simulink model "Capstone_MPC_Final"  (R2024b)
settings: Solver=ode4  StartTime=0.0  StopTime=tsim  FixedStep=baseRate  RelTol=1e-6  AbsTol=1e-6
values from neighbouring files (symbols this model uses):
  C = [cos(theta), -sin(theta) ... (first row only)    [Run_Initializer.m]
  docking_face = [0 1]'    [Run_Initializer.m]
  docking_offset = [0 0 0]'    [Run_Initializer.m]
  eta = 0.2    [Run_Initializer.m]
  F_t = [kron(eye(N_h),  [zeros(2,3), eye(2), zeros(2,4)]) ... (first row only)    [Run_Initializer.m]
  f_t = [kron(ones(N_h, 1), [xLength yLength]' - edge_buffer) ... (first row only)    [Run_Initializer.m]
  F_u = [kron(eye(N_h),  [eye(3), zeros(3,6)]) ... (first row only)    [Run_Initializer.m]
  f_u = kron(ones(2*N_h, 1), u_max')    [Run_Initializer.m]
  F_v = [kron(eye(N_h),  [zeros(1,5), 1, zeros(1,3)]) ... (first row only)    [Run_Initializer.m]
  gamma = 0.95    [Run_Initializer.m]
  Gamma1_el = 0.12    [Run_Initializer.m]
  Gamma1_sh = 0.005    [Run_Initializer.m]
  Gamma1_wr = 0.025    [Run_Initializer.m]
  Gamma2_el = 5    [Run_Initializer.m]
  Gamma2_sh = 5    [Run_Initializer.m]
  Gamma2_wr = 5    [Run_Initializer.m]
  Gamma3_el = 10    [Run_Initializer.m]
  Gamma3_sh = 40    [Run_Initializer.m]
  Gamma3_wr = 40    [Run_Initializer.m]
  Gamma4_el = 0.039    [Run_Initializer.m]
  Gamma4_sh = 0.015    [Run_Initializer.m]
  Gamma4_wr = 0.029    [Run_Initializer.m]
  Gamma5_el = 800    [Run_Initializer.m]
  Gamma5_sh = 800    [Run_Initializer.m]
  Gamma5_wr = 800    [Run_Initializer.m]
  Gamma6_el = 0.000001    (= 1e-06)    [Run_Initializer.m]
  Gamma6_sh = 0.005    [Run_Initializer.m]
  Gamma6_wr = 0.02    [Run_Initializer.m]
  H = kron(eye(N_h), [R, zeros(3,6); zeros(6,3), Q])    [Run_Initializer.m]
  Kd_elarm = 0.8    [Run_Initializer.m]
  Kd_sharm = 1.0    (= 1)    [Run_Initializer.m]
  Kd_wrarm = 0.6    [Run_Initializer.m]
  Kp_elarm = 1.2    [Run_Initializer.m]
  Kp_sharm = 1.5    [Run_Initializer.m]
  Kp_wrarm = 1.0    (= 1)    [Run_Initializer.m]
  lambda = (alpha^2)*(6 + kappa) - 6    (= 15.06)    [Run_Initializer.m]
  lidar_FOV = 40*d2r    (= 0.698131700798)    [Run_Initializer.m]
  lidar_offset = [0.145, 0.087]'    [Run_Initializer.m]
  PWMFreq = 5    [Run_Initializer.m]
  Q_k = [1e-6*eye(3)  zeros(3,3) ... (first row only)    [Run_Initializer.m]
  r_hold_min = [0.8; (0.3+0.05)]    [Run_Initializer.m]
  R_k = diag([0.02^2 0.02^2 0.01^2])    [Run_Initializer.m]
  T_d = 2    [Run_Initializer.m]
  Tz_lim_elarm = .1    (= 0.1)    [Run_Initializer.m]
  Tz_lim_sharm = .1    (= 0.1)    [Run_Initializer.m]
  Tz_lim_wrarm = .1    (= 0.1)    [Run_Initializer.m]
  w_c = [w_c0, w_i.*ones(1, 2*6)]    [Run_Initializer.m]
  w_m = [w_m0, w_i.*ones(1, 2*6)]    [Run_Initializer.m]
  x_BLACK_0 = [(1/3)*xLength (1/3)*yLength-0.2 280*d2r 0.01 0.005 1.88*d2r]'    [Run_Initializer.m]
  x_RED_0 = [3.2 2.1 0 0 0 0]'    [Run_Initializer.m]
  zeta = 10*d2r    (= 0.174532925199)    [Run_Initializer.m]
undefined symbols (not defined in the file or in its folder): a1, a2, a3, b0, b1, b2, b3, baseRate, dataRate, DiscIntNeverNeededParam, drop_states_ARM, drop_states_BLACK, drop_states_BLUE, drop_states_RED, F_black_X_nominal, F_black_Y_nominal, F_blue_X_nominal, F_blue_Y_nominal, F_red_X_nominal, F_red_Y_nominal, F_thrusters_BLACK, F_thrusters_BLUE, F_thrusters_RED, home_states_BLACK, home_states_BLUE, home_states_RED, IBLACK, IBLUE, IDIST, IEE, init_states_BLACK, init_states_BLUE, init_states_RED, IPROX, IRED, K_BLACK, K_BLUE, K_RED, Kd_tb, Kd_tblue, Kd_tr, Kd_xb, Kd_xblue, Kd_xr, Kd_yb, Kd_yblue, Kd_yr, Kp_tb, Kp_tblue, Kp_tr, Kp_xb, Kp_xblue, Kp_xr, Kp_yb, Kp_yblue, Kp_yr, mBLACK, mBLUE, mDIST, mEE ... (+21)
libraries: simulink x30, nvidiaSharedBlocks x18, MainLibrary x5, dspsigops x4, dspstat3 x3, dspinverses x3, dspmathops x1, nvidiaIMUSensorslib x1
(part 2 of 8)

== system Capstone_MPC_Final/Gyro.//Accel. Code ==
  Data Store Read1 : DataStoreRead  DataStoreName=isSim  IndexOptions=Index vector (dialog)  Indices=1  OutputSizes=1
  Log Gyro/Accel : Subsystem  TreatAsAtomicUnit=on
  This IF block determines whether or not to run the exp code : If  IfExpression=u1 == 0  ShowElse=off
  wires:
  This IF block determines whether or not to run the exp code/1 -> Log Gyro/Accel/Action
  Data Store Read1/1 -> This IF block determines whether or not to run the exp code/1

== system Capstone_MPC_Final/LiDAR Camera Code ==
  Check Measurement : MATLAB Function  TreatAsAtomicUnit=on
  Data Store Write : DataStoreWrite  DataStoreName=LiDAR_Data  IndexOptions=Index vector (dialog)  Indices=1  OutputSizes=1
  Data Type Conversion : DataTypeConversion  SaturateOnIntegerOverflow=off  RndMeth=Floor
  Delay : Delay  DelayLength=1  InitialCondition=0
  Demux : Demux  Outputs=[8,1]
  Equal : RelationalOperator  Operator=~=  OutDataTypeStr=boolean  RndMeth=Simplest  InputSameDT=off
  Get Real Measurement : Subsystem
  Get Simulated Measurement : Subsystem
  If : If
  Recieve Computer Vision Data : nvidiaSharedBlocks/UDP Receive  localURL='0.0.0.0'  localPort=43002  remoteURL='0.0.0.0'  remotePort=-1  recvBufferSize=8192  signalDatatype=single  dims=9  isVarSize=off  showBlockingTime=off  blockingTime=0  sampletime=-1  blockPlatform=NVIDIA
  Reshape : Reshape  OutputDimensionality=Customize  OutputDimensions=[9,1]
  Simulate Measurements : Constant  Value=0  OutDataTypeStr=Inherit: Inherit via back propagation
  Terminator : Terminator
  wires:
  If/1 -> Get Simulated Measurement/Action
  Simulate Measurements/1 -> If/1
  If/2 -> Get Real Measurement/Action
  Recieve Computer Vision Data/1 -> Data Type Conversion/1
  Data Type Conversion/1 -> Reshape/1
  Recieve Computer Vision Data/2 -> Terminator/1
  Equal/1 -> Check Measurement/2(new)
  Demux/1 -> Check Measurement/1("z ")
  Reshape/1 -> Demux/1
  Demux/2 -> Equal/2, Delay/1
  Delay/1 -> Equal/1
  Check Measurement/1(z) -> Data Store Write/1

== system Capstone_MPC_Final/Manipulator Encoder Data ==
  note: This if statement checks if a simulation is being performed. If not, it also checks that this code is being run on the RED platform. If it is, then the arm encoders are used to collect the joint angles. NOTE, the encoder data is collected very slowly, about 0.5 Hz. When the diagram is running faster then this collection rate, previous values of the encoder are held constant.
  Change ARM Behavior : Subsystem  TreatAsAtomicUnit=on
  Data Store Read1 : DataStoreRead  DataStoreName=WhoAmI  IndexOptions=Index vector (dialog)  Indices=1  OutputSizes=1
  Data Store Read2 : DataStoreRead  DataStoreName=isSim  IndexOptions=Index vector (dialog)  Indices=1  OutputSizes=1
  "This IF block determines whether or not to run the RED sim/exp " : If  NumInputs=2  IfExpression=u1 == 1 & u2 == 0  ShowElse=off
  wires:
  Data Store Read2/1 -> "This IF block determines whether or not to run the RED sim/exp "/2
  "This IF block determines whether or not to run the RED sim/exp "/1 -> Change ARM Behavior/Action
  Data Store Read1/1 -> "This IF block determines whether or not to run the RED sim/exp "/1

== system Capstone_MPC_Final/Model Predictive Control ==
  Enable : EnablePort
  Clock : Clock
  Data Store Write : DataStoreWrite  DataStoreName=Shutoff_Time  IndexOptions=Index vector (dialog)  Indices=1  OutputSizes=1
  Model Predictive Control : Subsystem  TreatAsAtomicUnit=on  SystemSampleTime=T_d
  Unscented Kalman Filter : Subsystem  TreatAsAtomicUnit=on  SystemSampleTime=baseRate
  wires:
  Clock/1 -> Data Store Write/1

== system Capstone_MPC_Final/PhaseSpace Camera Code ==
  note: In this subsection, the "if" statement is used to determine if this is a simulation or not. If it is not a simulation, then code is run to receive PhaseSpace camera data via UDP. The PhaseSpace code is currently a standalone executable that should not need to be modified by most users. The code sends all data for all platforms to each platform near simultaneously. If this is a simulation, then no data is required, but a continuous clock is created.
  Data Store Read2 : DataStoreRead  DataStoreName=isSim  IndexOptions=Index vector (dialog)  Indices=1  OutputSizes=1
  "If performing an experiment, grab the PhaseSpace data. Otherwise, use a clock to set time in SIM." : If  IfExpression=u1 == 0  ElseIfExpressions=u1 == 1  ShowElse=off
  Initialize Universal Time (Simulation) : Subsystem  TreatAsAtomicUnit=on
  Use Hardware to Obtain States : Subsystem  TreatAsAtomicUnit=on
  wires:
  Data Store Read2/1 -> "If performing an experiment, grab the PhaseSpace data. Otherwise, use a clock to set time in SIM."/1
  "If performing an experiment, grab the PhaseSpace data. Otherwise, use a clock to set time in SIM."/2 -> Initialize Universal Time (Simulation)/Action
  "If performing an experiment, grab the PhaseSpace data. Otherwise, use a clock to set time in SIM."/1 -> Use Hardware to Obtain States/Action

== system Capstone_MPC_Final/Platform Identification ==
  Data Store Read1 : DataStoreRead  DataStoreName=isSim  IndexOptions=Index vector (dialog)  Indices=1  OutputSizes=1
  "If 'simMode' set to '1', then this is a simulation and the dynamics will be simulated. Otherwise, this is an experiment, and the simulation will not be run." : If  IfExpression=u1 == 0  ShowElse=off
  Subsystem : Subsystem
  wires:
  "If 'simMode' set to '1', then this is a simulation and the dynamics will be simulated. Otherwise, this is an experiment, and the simulation will not be run."/1 -> Subsystem/Action
  Data Store Read1/1 -> "If 'simMode' set to '1', then this is a simulation and the dynamics will be simulated. Otherwise, this is an experiment, and the simulation will not be run."/1

== system Capstone_MPC_Final/Robotic Arm Code ==
  note: In this subsection, the "if" statements are used to determine two things: 1) whether or not a simulation is begin performed,
      | then 2) if an experiment is being performed, then which platform is the diagram compiled on. The "IdentifyPlatform" variable
      | is obtained using a custom C++ function which gets the computer name for each platform. NOTE that the arm code only runs on RED.
  Change ARM Behavior : Subsystem  TreatAsAtomicUnit=on
  Data Store Read : DataStoreRead  DataStoreName=WhoAmI  IndexOptions=Index vector (dialog)  Indices=1  OutputSizes=1
  Data Store Read1 : DataStoreRead  DataStoreName=isSim  IndexOptions=Index vector (dialog)  Indices=1  OutputSizes=1
  "This IF block determines whether or not to run the RED sim/exp " : If  NumInputs=2  IfExpression=u1 == 1 & u2 == 0  ShowElse=off
  wires:
  "This IF block determines whether or not to run the RED sim/exp "/1 -> Change ARM Behavior/Action
  Data Store Read1/1 -> "This IF block determines whether or not to run the RED sim/exp "/2
  Data Store Read/1 -> "This IF block determines whether or not to run the RED sim/exp "/1

== system Capstone_MPC_Final/Send Data to Orin ==
  Data Store Read1 : DataStoreRead  DataStoreName=isSim  IndexOptions=Index vector (dialog)  Indices=1  OutputSizes=1
  "If 'simMode' set to '1', then this is a simulation and the dynamics will be simulated. Otherwise, this is an experiment, and the simulation will not be run." : If  IfExpression=u1 == 0  ShowElse=off
  Subsystem : Subsystem
  wires:
  "If 'simMode' set to '1', then this is a simulation and the dynamics will be simulated. Otherwise, this is an experiment, and the simulation will not be run."/1 -> Subsystem/Action
  Data Store Read1/1 -> "If 'simMode' set to '1', then this is a simulation and the dynamics will be simulated. Otherwise, this is an experiment, and the simulation will not be run."/1

== system Capstone_MPC_Final/Simulate Plant Dynamics ==
  Action Port : ActionPort  ActionPortLabel=if(u1 == 1)
  BLACK Dynamics : Subsystem
  BLUE Dynamics : Subsystem
  RED and ARM Dynamics : Subsystem

== system Capstone_MPC_Final/Simulation Status ==
  Constant : Constant  Value=simMode  SampleTime=-1
  Data Store Write : DataStoreWrite  DataStoreName=isSim  IndexOptions=Index vector (dialog)  Indices=1  OutputSizes=1
  wires:
  Constant/1 -> Data Store Write/1

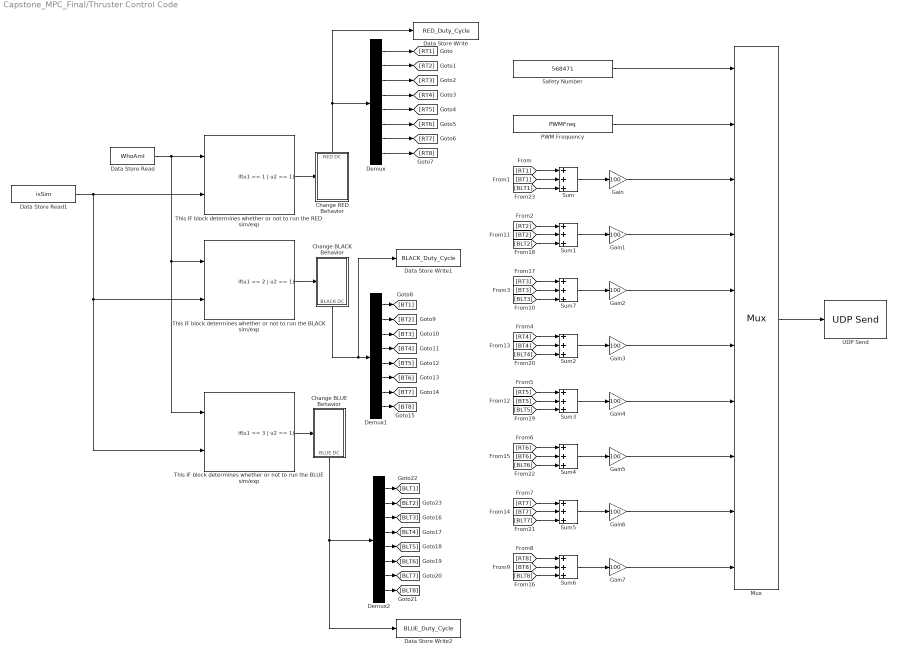
== system Capstone_MPC_Final/Thruster Control Code ==
  Change BLACK Behavior : Subsystem  TreatAsAtomicUnit=on
  Change BLUE Behavior : Subsystem  TreatAsAtomicUnit=on
  Change RED Behavior : Subsystem  TreatAsAtomicUnit=on
  Data Store Read : DataStoreRead  DataStoreName=WhoAmI  IndexOptions=Index vector (dialog)  Indices=1  OutputSizes=1
  Data Store Read1 : DataStoreRead  DataStoreName=isSim  IndexOptions=Index vector (dialog)  Indices=1  OutputSizes=1
  Data Store Write : DataStoreWrite  DataStoreName=RED_Duty_Cycle  IndexOptions=Index vector (dialog)  Indices=1  OutputSizes=1
  Data Store Write1 : DataStoreWrite  DataStoreName=BLACK_Duty_Cycle  IndexOptions=Index vector (dialog)  Indices=1  OutputSizes=1
  Data Store Write2 : DataStoreWrite  DataStoreName=BLUE_Duty_Cycle  IndexOptions=Index vector (dialog)  Indices=1  OutputSizes=1
  Demux : Demux  Outputs=8
  Demux1 : Demux  Outputs=8
  Demux2 : Demux  Outputs=8
  Gain{,1..7} (8 alike) : Gain  Gain=100
  Mux : Mux  Inputs=10
  PWM Frequency : Constant  Value=PWMFreq
  Safety Number : Constant  Value=568471
  Sum{,1..7} (8 alike) : Sum  Inputs=+++
  This IF block determines whether or not to run the BLACK sim/exp : If  NumInputs=2  IfExpression=u1 == 2 | u2 == 1  ShowElse=off
  This IF block determines whether or not to run the BLUE sim/exp : If  NumInputs=2  IfExpression=u1 == 3 | u2 == 1  ShowElse=off
  "This IF block determines whether or not to run the RED sim/exp " : If  NumInputs=2  IfExpression=u1 == 1 | u2 == 1  ShowElse=off
  UDP Send : nvidiaSharedBlocks/UDP Send  remoteURL='127.0.0.1'  remotePort=48291  localURL='0.0.0.0'  localPortSource=Automatically determine  localPort=-1  sampletime=-1  blockPlatform=NVIDIA  separateLengthPort=0
  wires:
  Data Store Read1/1 -> This IF block determines whether or not to run the BLACK sim/exp/2, This IF block determines whether or not to run the BLUE sim/exp/2, "This IF block determines whether or not to run the RED sim/exp "/2
  "This IF block determines whether or not to run the RED sim/exp "/1 -> Change RED Behavior/Action
  This IF block determines whether or not to run the BLACK sim/exp/1 -> Change BLACK Behavior/Action
  Change RED Behavior/1(RED DC) -> Demux/1, Data Store Write/1
  Demux/1 -> [RT1]
  Demux/2 -> [RT2]
  Demux/3 -> [RT3]
  Demux/4 -> [RT4]
  Demux/5 -> [RT5]
  Demux/6 -> [RT6]
  Demux/7 -> [RT7]
  Demux/8 -> [RT8]
  Demux1/5 -> [BT5]
  Demux1/4 -> [BT4]
  Demux1/1 -> [BT1]
  Demux1/8 -> [BT8]
  Demux1/2 -> [BT2]
  Demux1/7 -> [BT7]
  Demux1/6 -> [BT6]
  Demux1/3 -> [BT3]
  Change BLACK Behavior/1(BLACK DC) -> Demux1/1, Data Store Write1/1
  Data Store Read/1 -> This IF block determines whether or not to run the BLUE sim/exp/1, This IF block determines whether or not to run the BLACK sim/exp/1, "This IF block determines whether or not to run the RED sim/exp "/1
  This IF block determines whether or not to run the BLUE sim/exp/1 -> Change BLUE Behavior/Action
  Demux2/5 -> [BLT5]
  Demux2/8 -> [BLT8]
  Demux2/7 -> [BLT7]
  Demux2/2 -> [BLT2]
  Change BLUE Behavior/1(BLUE DC) -> Data Store Write2/1, Demux2/1
  Demux2/1 -> [BLT1]
  Demux2/4 -> [BLT4]
  Demux2/3 -> [BLT3]
  Demux2/6 -> [BLT6]
  [BT5] -> Sum3/2
  [RT4] -> Sum2/1
  Sum3/1 -> Gain4/1
  [RT2] -> Sum1/1
  [BLT4] -> Sum2/3
  [BT3] -> Sum7/2
  [RT5] -> Sum3/1
  PWM Frequency/1 -> Mux/2
  Gain3/1 -> Mux/6
  [BT8] -> Sum6/2
  Gain7/1 -> Mux/10
  Sum6/1 -> Gain7/1
  Sum7/1 -> Gain2/1
  [BT4] -> Sum2/2
  [RT7] -> Sum5/1
  [BLT3] -> Sum7/3
  Gain1/1 -> Mux/4
  Gain/1 -> Mux/3
  [BLT5] -> Sum3/3
  Sum1/1 -> Gain1/1
  Sum2/1 -> Gain3/1
  Gain4/1 -> Mux/7
  [BLT6] -> Sum4/3
  [BT6] -> Sum4/2
  [BT2] -> Sum1/2
  [BLT2] -> Sum1/3
  [RT1] -> Sum/1
  Sum/1 -> Gain/1
  [BT7] -> Sum5/2
  Gain6/1 -> Mux/9
  [BLT7] -> Sum5/3
  [RT8] -> Sum6/1
  [RT6] -> Sum4/1
  Mux/1 -> UDP Send/1
  [BLT8] -> Sum6/3
  [BT1] -> Sum/2
  Sum5/1 -> Gain6/1
  Gain5/1 -> Mux/8
  Sum4/1 -> Gain5/1
  [BLT1] -> Sum/3
  Safety Number/1 -> Mux/1
  [RT3] -> Sum7/1
  Gain2/1 -> Mux/5

== system Capstone_MPC_Final/1 - Experiment Logic/Phase #0: Synchronization ==
  note: Setting the RED thrusters to OFF.
  note: Setting the PUCKS for ALL to OFF.
  note: DISABLE ARM Path Planning.
  note: Setting the BLACK thrusters to OFF.
  note: Setting the BLUE thrusters to OFF.
  note: DISABLE RED Path Planning.
  note: DISABLE BLACK Path Planning.
  note: DISABLE BLUE Path Planning.
  note: DISABLE ARM Control.
  Action Port : ActionPort  ActionPortLabel=if(u1 < u2)
  Constant{1..8} (8 alike) : Constant  Value=0
  Data Store Write : DataStoreWrite  DataStoreName=RED_Control_Law_Enabler  IndexOptions=Index vector (dialog)  Indices=1  OutputSizes=1
  Data Store Write1 : DataStoreWrite  DataStoreName=RED_Logger  IndexOptions=Index vector (dialog)  Indices=1  OutputSizes=1
  Data Store Write2 : DataStoreWrite  DataStoreName=BLACK_Control_Law_Enabler  IndexOptions=Index vector (dialog)  Indices=1  OutputSizes=1
  Data Store Write3 : DataStoreWrite  DataStoreName=BLUE_Control_Law_Enabler  IndexOptions=Index vector (dialog)  Indices=1  OutputSizes=1
  Data Store Write4 : DataStoreWrite  DataStoreName=Float_State  IndexOptions=Index vector (dialog)  Indices=1  OutputSizes=1
  Data Store Write5 : DataStoreWrite  DataStoreName=BLUE_Path_Planner_Selection  IndexOptions=Index vector (dialog)  Indices=1  OutputSizes=1
  Data Store Write6 : DataStoreWrite  DataStoreName=BLACK_Path_Planner_Selection  IndexOptions=Index vector (dialog)  Indices=1  OutputSizes=1
  Data Store Write7 : DataStoreWrite  DataStoreName=RED_Path_Planner_Selection  IndexOptions=Index vector (dialog)  Indices=1  OutputSizes=1
  Data Store Write8 : DataStoreWrite  DataStoreName=ARM_Path_Planner_Selection  IndexOptions=Index vector (dialog)  Indices=1  OutputSizes=1
  Data Store Write9 : DataStoreWrite  DataStoreName=ARM_Control_Law_Enabler  IndexOptions=Index vector (dialog)  Indices=1  OutputSizes=1
  Puck State : Constant  Value=0
  String Constant : StringConstant  String="\"Chaser: Running Phase 0\""
  wires:
  Constant4/1 -> Data Store Write8/1
  Puck State/1 -> Data Store Write4/1
  Constant5/1 -> Data Store Write/1
  Constant1/1 -> Data Store Write2/1
  Constant2/1 -> Data Store Write3/1
  Constant3/1 -> Data Store Write7/1
  Constant6/1 -> Data Store Write6/1
  Constant7/1 -> Data Store Write5/1
  Constant8/1 -> Data Store Write9/1
  String Constant/1 -> Data Store Write1/1

== system Capstone_MPC_Final/1 - Experiment Logic/Phase #1: Start Floating  ==
  note: DISABLE ARM Control.
  note: Setting the BLACK thrusters to OFF.
  note: Setting the PUCKS for ALL to OFF.
  note: DISABLE RED Path Planning.
  note: Setting the RED thrusters to OFF.
  note: Setting the BLUE thrusters to OFF.
  note: DISABLE ARM Path Planning.
  note: DISABLE BLACK Path Planning.
  note: DISABLE BLUE Path Planning.
  Action Port : ActionPort  ActionPortLabel=elseif((u1 < u3 & u1 >= u2))
  Constant{1..8} (8 alike) : Constant  Value=0
  Data Store Write : DataStoreWrite  DataStoreName=RED_Control_Law_Enabler  IndexOptions=Index vector (dialog)  Indices=1  OutputSizes=1
  Data Store Write1 : DataStoreWrite  DataStoreName=RED_Logger  IndexOptions=Index vector (dialog)  Indices=1  OutputSizes=1
  Data Store Write2 : DataStoreWrite  DataStoreName=BLACK_Control_Law_Enabler  IndexOptions=Index vector (dialog)  Indices=1  OutputSizes=1
  Data Store Write3 : DataStoreWrite  DataStoreName=BLUE_Control_Law_Enabler  IndexOptions=Index vector (dialog)  Indices=1  OutputSizes=1
  Data Store Write4 : DataStoreWrite  DataStoreName=Float_State  IndexOptions=Index vector (dialog)  Indices=1  OutputSizes=1
  Data Store Write5 : DataStoreWrite  DataStoreName=BLUE_Path_Planner_Selection  IndexOptions=Index vector (dialog)  Indices=1  OutputSizes=1
  Data Store Write6 : DataStoreWrite  DataStoreName=BLACK_Path_Planner_Selection  IndexOptions=Index vector (dialog)  Indices=1  OutputSizes=1
  Data Store Write7 : DataStoreWrite  DataStoreName=RED_Path_Planner_Selection  IndexOptions=Index vector (dialog)  Indices=1  OutputSizes=1
  Data Store Write8 : DataStoreWrite  DataStoreName=ARM_Path_Planner_Selection  IndexOptions=Index vector (dialog)  Indices=1  OutputSizes=1
  Data Store Write9 : DataStoreWrite  DataStoreName=ARM_Control_Law_Enabler  IndexOptions=Index vector (dialog)  Indices=1  OutputSizes=1
  Puck State : Constant
  String Constant : StringConstant  String="\"Chaser: Running Phase 1\""
  wires:
  Constant7/1 -> Data Store Write5/1
  Constant2/1 -> Data Store Write3/1
  Constant6/1 -> Data Store Write6/1
  Puck State/1 -> Data Store Write4/1
  Constant1/1 -> Data Store Write2/1
  Constant5/1 -> Data Store Write/1
  Constant3/1 -> Data Store Write7/1
  Constant8/1 -> Data Store Write9/1
  Constant4/1 -> Data Store Write8/1
  String Constant/1 -> Data Store Write1/1

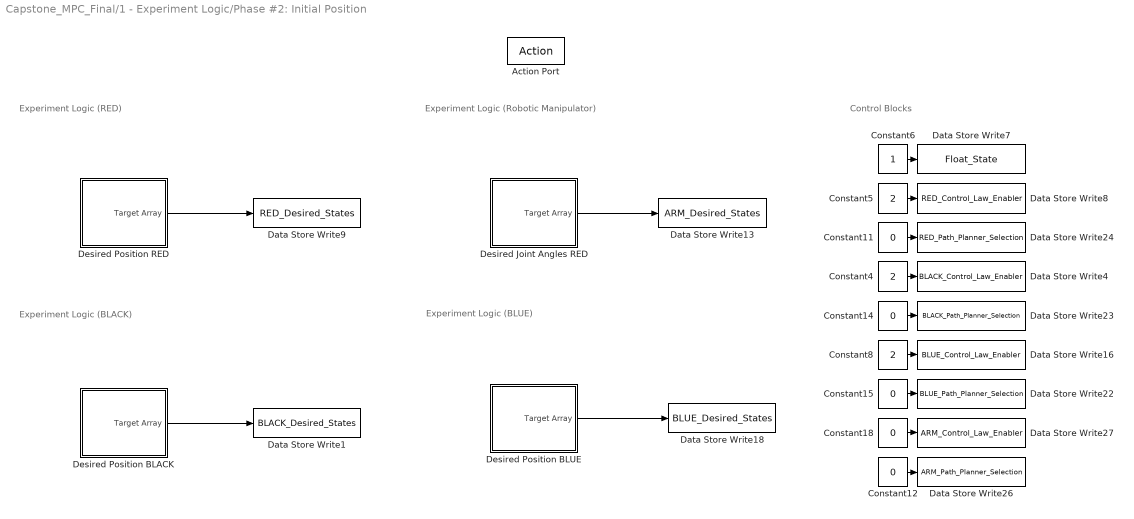
== system Capstone_MPC_Final/1 - Experiment Logic/Phase #2: Initial Position ==
  note: Experiment Logic (BLACK)
  note: Control Blocks
  note: Experiment Logic (RED)
  note: Experiment Logic (Robotic Manipulator)
  note: Experiment Logic (BLUE)
  Action Port : ActionPort  ActionPortLabel=elseif((u1 < u4 & u1 >= u3))
  Constant{11..12,14..15,18} (5 alike) : Constant  Value=0
  Constant4 : Constant  Value=2
  Constant5 : Constant  Value=2
  Constant6 : Constant
  Constant8 : Constant  Value=2
  Data Store Write1 : DataStoreWrite  DataStoreName=BLACK_Desired_States  IndexOptions=Index vector (dialog)  Indices=1  OutputSizes=1
  Data Store Write13 : DataStoreWrite  DataStoreName=ARM_Desired_States  IndexOptions=Index vector (dialog)  Indices=1  OutputSizes=1
  Data Store Write16 : DataStoreWrite  DataStoreName=BLUE_Control_Law_Enabler  IndexOptions=Index vector (dialog)  Indices=1  OutputSizes=1
  Data Store Write18 : DataStoreWrite  DataStoreName=BLUE_Desired_States  IndexOptions=Index vector (dialog)  Indices=1  OutputSizes=1
  Data Store Write22 : DataStoreWrite  DataStoreName=BLUE_Path_Planner_Selection  IndexOptions=Index vector (dialog)  Indices=1  OutputSizes=1
  Data Store Write23 : DataStoreWrite  DataStoreName=BLACK_Path_Planner_Selection  IndexOptions=Index vector (dialog)  Indices=1  OutputSizes=1
  Data Store Write24 : DataStoreWrite  DataStoreName=RED_Path_Planner_Selection  IndexOptions=Index vector (dialog)  Indices=1  OutputSizes=1
  Data Store Write26 : DataStoreWrite  DataStoreName=ARM_Path_Planner_Selection  IndexOptions=Index vector (dialog)  Indices=1  OutputSizes=1
  Data Store Write27 : DataStoreWrite  DataStoreName=ARM_Control_Law_Enabler  IndexOptions=Index vector (dialog)  Indices=1  OutputSizes=1
  Data Store Write4 : DataStoreWrite  DataStoreName=BLACK_Control_Law_Enabler  IndexOptions=Index vector (dialog)  Indices=1  OutputSizes=1
  Data Store Write7 : DataStoreWrite  DataStoreName=Float_State  IndexOptions=Index vector (dialog)  Indices=1  OutputSizes=1
  Data Store Write8 : DataStoreWrite  DataStoreName=RED_Control_Law_Enabler  IndexOptions=Index vector (dialog)  Indices=1  OutputSizes=1
  Data Store Write9 : DataStoreWrite  DataStoreName=RED_Desired_States  IndexOptions=Index vector (dialog)  Indices=1  OutputSizes=1
  Desired Joint Angles RED : Subsystem
  Desired Position BLACK : Subsystem
  Desired Position BLUE : Subsystem
  Desired Position RED : Subsystem
  wires:
  Constant4/1 -> Data Store Write4/1
  Constant8/1 -> Data Store Write16/1
  Desired Position BLACK/1(Target Array) -> Data Store Write1/1
  Constant5/1 -> Data Store Write8/1
  Desired Position RED/1(Target Array) -> Data Store Write9/1
  Constant6/1 -> Data Store Write7/1
  Desired Position BLUE/1(Target Array) -> Data Store Write18/1
  Constant11/1 -> Data Store Write24/1
  Constant14/1 -> Data Store Write23/1
  Constant15/1 -> Data Store Write22/1
  Desired Joint Angles RED/1(Target Array) -> Data Store Write13/1
  Constant18/1 -> Data Store Write27/1
  Constant12/1 -> Data Store Write26/1

== system Capstone_MPC_Final/1 - Experiment Logic/Phase #3: Experiment ==
  Action Port : ActionPort  ActionPortLabel=elseif( (u1 < u5 & u1 >= u4))
  Constant1 : Constant  Value=Phase3_SubPhase2_End  SampleTime=-1
  Constant2 : Constant  Value=Phase3_SubPhase3_End  SampleTime=-1
  Constant3 : Constant  Value=Phase3_SubPhase4_End  SampleTime=-1
  Constant4 : Constant  Value=Phase3_SubPhase1_End  SampleTime=-1
  Experiment Sub-Phases : If  NumInputs=5  IfExpression=u1 < u2  ElseIfExpressions=(u1 < u3 & u1 >= u2),(u1 < u4 & u1 >= u3), (u1 < u5 & u1 >= u4)  ShowElse=off
  Sub-Phase #1 : Subsystem  TreatAsAtomicUnit=on
  Sub-Phase #2 : Subsystem  TreatAsAtomicUnit=on
  Sub-Phase #3 : Subsystem  TreatAsAtomicUnit=on
  Sub-Phase #4 : Subsystem  TreatAsAtomicUnit=on
  Universal_Time : DataStoreRead  DataStoreName=Univ_Time  IndexOptions=Index vector (dialog)  Indices=1  OutputSizes=1
  wires:
  Experiment Sub-Phases/3 -> Sub-Phase #3/Action
  Experiment Sub-Phases/4 -> Sub-Phase #4/Action
  Constant3/1 -> Experiment Sub-Phases/5
  Constant2/1 -> Experiment Sub-Phases/4
  Experiment Sub-Phases/1 -> Sub-Phase #1/Action
  Experiment Sub-Phases/2 -> Sub-Phase #2/Action
  Constant1/1 -> Experiment Sub-Phases/3
  Constant4/1 -> Experiment Sub-Phases/2
  Universal_Time/1 -> Experiment Sub-Phases/1

== system Capstone_MPC_Final/1 - Experiment Logic/Phase #4: Return Home ==
  note: Experiment Logic (BLACK)
  note: Experiment Logic (Robotic Manipulator)
  note: Experiment Logic (BLUE)
  note: Experiment Logic (RED)
  note: Control Blocks
  Action Port : ActionPort  ActionPortLabel=elseif((u1 < u6 & u1 >= u5))
  Constant{11..12,14..15,18} (5 alike) : Constant  Value=0
  Constant4 : Constant  Value=2
  Constant5 : Constant  Value=2
  Constant6 : Constant
  Constant8 : Constant  Value=2
  Data Store Write13 : DataStoreWrite  DataStoreName=ARM_Desired_States  IndexOptions=Index vector (dialog)  Indices=1  OutputSizes=1
  Data Store Write16 : DataStoreWrite  DataStoreName=BLUE_Control_Law_Enabler  IndexOptions=Index vector (dialog)  Indices=1  OutputSizes=1
  Data Store Write18 : DataStoreWrite  DataStoreName=BLUE_Desired_States  IndexOptions=Index vector (dialog)  Indices=1  OutputSizes=1
  Data Store Write22 : DataStoreWrite  DataStoreName=BLUE_Path_Planner_Selection  IndexOptions=Index vector (dialog)  Indices=1  OutputSizes=1
  Data Store Write23 : DataStoreWrite  DataStoreName=BLACK_Path_Planner_Selection  IndexOptions=Index vector (dialog)  Indices=1  OutputSizes=1
  Data Store Write24 : DataStoreWrite  DataStoreName=RED_Path_Planner_Selection  IndexOptions=Index vector (dialog)  Indices=1  OutputSizes=1
  Data Store Write3 : DataStoreWrite  DataStoreName=ARM_Path_Planner_Selection  IndexOptions=Index vector (dialog)  Indices=1  OutputSizes=1
  Data Store Write4 : DataStoreWrite  DataStoreName=ARM_Control_Law_Enabler  IndexOptions=Index vector (dialog)  Indices=1  OutputSizes=1
  Data Store Write5 : DataStoreWrite  DataStoreName=BLACK_Control_Law_Enabler  IndexOptions=Index vector (dialog)  Indices=1  OutputSizes=1
  Data Store Write6 : DataStoreWrite  DataStoreName=BLACK_Desired_States  IndexOptions=Index vector (dialog)  Indices=1  OutputSizes=1
  Data Store Write7 : DataStoreWrite  DataStoreName=Float_State  IndexOptions=Index vector (dialog)  Indices=1  OutputSizes=1
  Data Store Write8 : DataStoreWrite  DataStoreName=RED_Control_Law_Enabler  IndexOptions=Index vector (dialog)  Indices=1  OutputSizes=1
  Data Store Write9 : DataStoreWrite  DataStoreName=RED_Desired_States  IndexOptions=Index vector (dialog)  Indices=1  OutputSizes=1
  Desired Joint Angles RED : Subsystem
  Desired Position BLACK : Subsystem
  Desired Position BLUE : Subsystem
  Desired Position RED : Subsystem
  wires:
  Desired Position RED/1(Target Array) -> Data Store Write9/1
  Desired Position BLACK/1(Target Array) -> Data Store Write6/1
  Desired Position BLUE/1(Target Array) -> Data Store Write18/1
  Constant12/1 -> Data Store Write3/1
  Constant18/1 -> Data Store Write4/1
  Constant6/1 -> Data Store Write7/1
  Constant15/1 -> Data Store Write22/1
  Constant14/1 -> Data Store Write23/1
  Constant5/1 -> Data Store Write8/1
  Constant11/1 -> Data Store Write24/1
  Constant8/1 -> Data Store Write16/1
  Constant4/1 -> Data Store Write5/1
  Desired Joint Angles RED/1(Target Array) -> Data Store Write13/1

== system Capstone_MPC_Final/1 - Experiment Logic/Phase #5: Hold Home ==
  note: Experiment Logic (BLUE)
  note: Experiment Logic (BLACK)
  note: Control Blocks
  note: Experiment Logic (RED)
  note: Experiment Logic (Robotic Manipulator)
  Action Port : ActionPort  ActionPortLabel=elseif( (u1 < u7 & u1 >= u6) )
  Constant{11..12,14..15,18} (5 alike) : Constant  Value=0
  Constant4 : Constant  Value=2
  Constant5 : Constant  Value=2
  Constant6 : Constant
  Constant8 : Constant  Value=2
  Data Store Write13 : DataStoreWrite  DataStoreName=ARM_Desired_States  IndexOptions=Index vector (dialog)  Indices=1  OutputSizes=1
  Data Store Write16 : DataStoreWrite  DataStoreName=BLUE_Control_Law_Enabler  IndexOptions=Index vector (dialog)  Indices=1  OutputSizes=1
  Data Store Write18 : DataStoreWrite  DataStoreName=BLUE_Desired_States  IndexOptions=Index vector (dialog)  Indices=1  OutputSizes=1
  Data Store Write22 : DataStoreWrite  DataStoreName=BLUE_Path_Planner_Selection  IndexOptions=Index vector (dialog)  Indices=1  OutputSizes=1
  Data Store Write23 : DataStoreWrite  DataStoreName=BLACK_Path_Planner_Selection  IndexOptions=Index vector (dialog)  Indices=1  OutputSizes=1
  Data Store Write24 : DataStoreWrite  DataStoreName=RED_Path_Planner_Selection  IndexOptions=Index vector (dialog)  Indices=1  OutputSizes=1
  Data Store Write3 : DataStoreWrite  DataStoreName=ARM_Path_Planner_Selection  IndexOptions=Index vector (dialog)  Indices=1  OutputSizes=1
  Data Store Write4 : DataStoreWrite  DataStoreName=ARM_Control_Law_Enabler  IndexOptions=Index vector (dialog)  Indices=1  OutputSizes=1
  Data Store Write5 : DataStoreWrite  DataStoreName=BLACK_Control_Law_Enabler  IndexOptions=Index vector (dialog)  Indices=1  OutputSizes=1
  Data Store Write6 : DataStoreWrite  DataStoreName=BLACK_Desired_States  IndexOptions=Index vector (dialog)  Indices=1  OutputSizes=1
  Data Store Write7 : DataStoreWrite  DataStoreName=Float_State  IndexOptions=Index vector (dialog)  Indices=1  OutputSizes=1
  Data Store Write8 : DataStoreWrite  DataStoreName=RED_Control_Law_Enabler  IndexOptions=Index vector (dialog)  Indices=1  OutputSizes=1
  Data Store Write9 : DataStoreWrite  DataStoreName=RED_Desired_States  IndexOptions=Index vector (dialog)  Indices=1  OutputSizes=1
  Desired Joint Angles RED : Subsystem
  Desired Position BLACK : Subsystem
  Desired Position BLUE : Subsystem
  Desired Position RED : Subsystem
  wires:
  Desired Position RED/1(Target Array) -> Data Store Write9/1
  Desired Position BLACK/1(Target Array) -> Data Store Write6/1
  Desired Position BLUE/1(Target Array) -> Data Store Write18/1
  Constant12/1 -> Data Store Write3/1
  Constant18/1 -> Data Store Write4/1
  Constant6/1 -> Data Store Write7/1
  Constant15/1 -> Data Store Write22/1
  Constant14/1 -> Data Store Write23/1
  Constant5/1 -> Data Store Write8/1
  Constant11/1 -> Data Store Write24/1
  Constant8/1 -> Data Store Write16/1
  Constant4/1 -> Data Store Write5/1
  Desired Joint Angles RED/1(Target Array) -> Data Store Write13/1

== system Capstone_MPC_Final/1 - Experiment Logic/Phase #6: Clean Shutdown ==
  note: DISABLE ARM Control.
  note: Setting the BLACK thrusters to OFF.
  note: Setting the PUCKS for ALL to OFF.
  note: DISABLE RED Path Planning.
  note: Setting the RED thrusters to OFF.
  note: Setting the BLUE thrusters to OFF.
  note: DISABLE ARM Path Planning.
  note: DISABLE BLACK Path Planning.
  note: DISABLE BLUE Path Planning.
  Action Port : ActionPort  ActionPortLabel=elseif((u1 >= u7))
  Constant{1..8} (8 alike) : Constant  Value=0
  Data Store Write : DataStoreWrite  DataStoreName=RED_Control_Law_Enabler  IndexOptions=Index vector (dialog)  Indices=1  OutputSizes=1
  Data Store Write2 : DataStoreWrite  DataStoreName=BLACK_Control_Law_Enabler  IndexOptions=Index vector (dialog)  Indices=1  OutputSizes=1
  Data Store Write3 : DataStoreWrite  DataStoreName=BLUE_Control_Law_Enabler  IndexOptions=Index vector (dialog)  Indices=1  OutputSizes=1
  Data Store Write4 : DataStoreWrite  DataStoreName=Float_State  IndexOptions=Index vector (dialog)  Indices=1  OutputSizes=1
  Data Store Write5 : DataStoreWrite  DataStoreName=BLUE_Path_Planner_Selection  IndexOptions=Index vector (dialog)  Indices=1  OutputSizes=1
  Data Store Write6 : DataStoreWrite  DataStoreName=BLACK_Path_Planner_Selection  IndexOptions=Index vector (dialog)  Indices=1  OutputSizes=1
  Data Store Write7 : DataStoreWrite  DataStoreName=RED_Path_Planner_Selection  IndexOptions=Index vector (dialog)  Indices=1  OutputSizes=1
  Data Store Write8 : DataStoreWrite  DataStoreName=ARM_Path_Planner_Selection  IndexOptions=Index vector (dialog)  Indices=1  OutputSizes=1
  Data Store Write9 : DataStoreWrite  DataStoreName=ARM_Control_Law_Enabler  IndexOptions=Index vector (dialog)  Indices=1  OutputSizes=1
  Puck State : Constant  Value=0
  wires:
  Constant7/1 -> Data Store Write5/1
  Constant2/1 -> Data Store Write3/1
  Constant6/1 -> Data Store Write6/1
  Puck State/1 -> Data Store Write4/1
  Constant1/1 -> Data Store Write2/1
  Constant5/1 -> Data Store Write/1
  Constant3/1 -> Data Store Write7/1
  Constant8/1 -> Data Store Write9/1
  Constant4/1 -> Data Store Write8/1

== system Capstone_MPC_Final/2 - Guidance/Custom PPL (ARM) ==
  Action Port : ActionPort  ActionPortLabel=if(u1 == 2)
  Desired Position : Subsystem
  Path : Outport
  wires:
  Desired Position/1(Position Array) -> Path/1

== system Capstone_MPC_Final/2 - Guidance/Custom PPL (BLACK) ==
  Action Port : ActionPort  ActionPortLabel=elseif(u1 == 2)
  Desired Position : Subsystem
  Path : Outport
  wires:
  Desired Position/1(Position Array) -> Path/1

== system Capstone_MPC_Final/2 - Guidance/Custom PPL (BLUE) ==
  Action Port : ActionPort  ActionPortLabel=if(u1 == 2)
  Desired Position : Subsystem
  Path : Outport
  wires:
  Desired Position/1(Position Array) -> Path/1

== system Capstone_MPC_Final/2 - Guidance/Custom PPL (RED) ==
  Action Port : ActionPort  ActionPortLabel=elseif(u1 == 2)
  Desired Position : Subsystem
  Path : Outport
  wires:
  Desired Position/1(Position Array) -> Path/1

== system Capstone_MPC_Final/2 - Guidance/Default APF PPL (BLACK) ==
  Action Port : ActionPort  ActionPortLabel=if(u1 == 1 )
  Angular Gain : Constant  Value=200
  Attractive Gain : Constant  Value=200
  Current Position RED : Subsystem
  Influence Range : Constant
  MATLAB Function : MATLAB Function  TreatAsAtomicUnit=on
  Obstacles : Subsystem
  RED_Px : DataStoreRead  DataStoreName=BLACK_Desired_States  IndexOptions=Index vector (dialog)  Indices=1  OutputSizes=1
  Repulsive Gain : Constant  Value=5
  Reshape : Reshape  OutputDimensionality=Row vector (2-D)
  Reshape1 : Reshape  OutputDimensionality=Row vector (2-D)
  Path : Outport
  wires:
  Obstacles/1(Obstacle Positions) -> MATLAB Function/3(obstacles)
  MATLAB Function/1(currentPosition) -> Path/1
  Reshape/1 -> MATLAB Function/1(desiredPosition)
  Angular Gain/1 -> MATLAB Function/7(angularGain)
  RED_Px/1 -> Reshape/1
  Attractive Gain/1 -> MATLAB Function/4(attractiveGain)
  Repulsive Gain/1 -> MATLAB Function/5(repulsiveGain)
  Reshape1/1 -> MATLAB Function/2("currentPosition ")
  Influence Range/1 -> MATLAB Function/6(influenceRange)
  Current Position RED/1(Position Array) -> Reshape1/1

== system Capstone_MPC_Final/2 - Guidance/Default APF PPL (RED) ==
  Action Port : ActionPort  ActionPortLabel=if(u1 == 1 )
  Angular Gain : Constant  Value=200
  Attractive Gain : Constant  Value=200
  Current Position RED : Subsystem
  Influence Range : Constant
  MATLAB Function : MATLAB Function  TreatAsAtomicUnit=on
  Obstacles : Subsystem
  RED_Px : DataStoreRead  DataStoreName=RED_Desired_States  IndexOptions=Index vector (dialog)  Indices=1  OutputSizes=1
  Repulsive Gain : Constant  Value=5
  Reshape : Reshape  OutputDimensionality=Row vector (2-D)
  Reshape1 : Reshape  OutputDimensionality=Row vector (2-D)
  Path : Outport
  wires:
  MATLAB Function/1(currentPosition) -> Path/1
  Reshape/1 -> MATLAB Function/1(desiredPosition)
  Reshape1/1 -> MATLAB Function/2("currentPosition ")
  Current Position RED/1(Position Array) -> Reshape1/1
  Obstacles/1(Obstacle Positions) -> MATLAB Function/3(obstacles)
  RED_Px/1 -> Reshape/1
  Attractive Gain/1 -> MATLAB Function/4(attractiveGain)
  Angular Gain/1 -> MATLAB Function/7(angularGain)
  Influence Range/1 -> MATLAB Function/6(influenceRange)
  Repulsive Gain/1 -> MATLAB Function/5(repulsiveGain)

== system Capstone_MPC_Final/2 - Guidance/Disable PPL (ARM) ==
  Action Port : ActionPort  ActionPortLabel=else
  Desired Position : Subsystem
  Path : Outport
  wires:
  Desired Position/1(Position Array) -> Path/1

== system Capstone_MPC_Final/2 - Guidance/Disable PPL (BLACK) ==
  Action Port : ActionPort  ActionPortLabel=else
  Desired Position : Subsystem
  Path : Outport
  wires:
  Desired Position/1(Position Array) -> Path/1

== system Capstone_MPC_Final/2 - Guidance/Disable PPL (BLUE) ==
  Action Port : ActionPort  ActionPortLabel=else
  Desired Position : Subsystem
  Path : Outport
  wires:
  Desired Position/1(Position Array) -> Path/1

== system Capstone_MPC_Final/2 - Guidance/Disable PPL (RED) ==
  Action Port : ActionPort  ActionPortLabel=else
  Desired Position : Subsystem
  Path : Outport
  wires:
  Desired Position/1(Position Array) -> Path/1

== system Capstone_MPC_Final/3 - Control/Custom Control (ARM) ==
  Action Port : ActionPort  ActionPortLabel=elseif(u1 == 2)
  Mux : Mux  Inputs=3
  Zero : Constant  Value=0  OutDataTypeStr=Inherit: Inherit via back propagation
  u : Outport
  wires:
  Mux/1 -> u/1
  Zero/1 -> Mux/3, Mux/1, Mux/2

== system Capstone_MPC_Final/3 - Control/Default LQR Control (BLACK) ==
  Action Port : ActionPort  ActionPortLabel=elseif(u1 == 2)
  Calculate Error : Subsystem
  Constant2 : Constant  Value=-K_BLACK
  Data Store Read1 : DataStoreRead  DataStoreName=BLACK_Path  IndexOptions=Index vector (dialog)  Indices=1  OutputSizes=1
  Data Store Read13 : DataStoreRead  DataStoreName=BLACK_Measured_States  IndexOptions=Index vector (dialog)  Indices=1  OutputSizes=1
  Demux : Demux  Outputs=[1,1,1,1,1,1,3]
  Demux1 : Demux  Outputs=3
  Discrete Derivative : simulink/Discrete/Discrete Derivative  gainval=1.0  ICPrevScaledInput=0.0  OutMin=[]  OutMax=[]  OutDataType=fixdt(1, 16)  OutScaling=2^-10  DoSatur=off
  Discrete Derivative1 : simulink/Discrete/Discrete Derivative  gainval=1.0  ICPrevScaledInput=0.0  OutMin=[]  OutMax=[]  OutDataType=fixdt(1, 16)  OutScaling=2^-10  DoSatur=off
  Discrete Derivative2 : simulink/Discrete/Discrete Derivative  gainval=1.0  ICPrevScaledInput=0.0  OutMin=[]  OutMax=[]  OutDataType=fixdt(1, 16)  OutScaling=2^-10  DoSatur=off
  Matrix Multiply : Product  Multiplication=Matrix(*)
  Mux1 : Mux  Inputs=3
  Mux2 : Mux  Inputs=2
  Mux3 : Mux  Inputs=3
  Reshape1 : Reshape  OutputDimensionality=Column vector (2-D)
  Reshape3 : Reshape  OutputDimensionality=Column vector (2-D)
  Reshape4 : Reshape  OutputDimensionality=Column vector (2-D)
  Subtract{4..8} (5 alike) : Sum  Inputs=-+
  Terminator : Terminator
  u : Outport
  wires:
  Mux2/1 -> Matrix Multiply/2
  Reshape1/1 -> Mux2/1
  Mux1/1 -> Reshape1/1
  Reshape3/1 -> Mux2/2
  Reshape4/1 -> u/1
  Matrix Multiply/1 -> Reshape4/1
  Constant2/1 -> Matrix Multiply/1
  Mux3/1 -> Reshape3/1
  Demux1/2 -> Discrete Derivative1/1, Subtract4/1
  Demux/2 -> Subtract4/2
  Demux1/3 -> Calculate Error/1(Desired Attitude), Discrete Derivative2/1
  Discrete Derivative1/1 -> Subtract6/1
  Demux/4 -> Subtract7/2
  Data Store Read13/1 -> Demux/1
  Demux/1 -> Subtract5/2
  Discrete Derivative/1 -> Subtract7/1
  Data Store Read1/1 -> Demux1/1
  Demux/5 -> Subtract6/2
  Demux/3 -> Calculate Error/2(Measured Attitude)
  Demux/7 -> Terminator/1
  Discrete Derivative2/1 -> Subtract8/1
  Demux1/1 -> Discrete Derivative/1, Subtract5/1
  Demux/6 -> Subtract8/2
  Subtract5/1 -> Mux1/1
  Subtract4/1 -> Mux1/2
  Calculate Error/1(Attitude Error) -> Mux1/3
  Subtract7/1 -> Mux3/1
  Subtract6/1 -> Mux3/2
  Subtract8/1 -> Mux3/3

== system Capstone_MPC_Final/3 - Control/Default LQR Control (BLUE) ==
  Action Port : ActionPort  ActionPortLabel=elseif(u1 == 2)
  Calculate Error : Subsystem
  Constant2 : Constant  Value=-K_BLUE
  Data Store Read1 : DataStoreRead  DataStoreName=BLUE_Path  IndexOptions=Index vector (dialog)  Indices=1  OutputSizes=1
  Data Store Read2 : DataStoreRead  DataStoreName=BLUE_Measured_States  IndexOptions=Index vector (dialog)  Indices=1  OutputSizes=1
  Demux : Demux  Outputs=[1,1,1,1,1,1,3]
  Demux1 : Demux  Outputs=3
  Discrete Derivative : simulink/Discrete/Discrete Derivative  gainval=1.0  ICPrevScaledInput=0.0  OutMin=[]  OutMax=[]  OutDataType=fixdt(1, 16)  OutScaling=2^-10  DoSatur=off
  Discrete Derivative1 : simulink/Discrete/Discrete Derivative  gainval=1.0  ICPrevScaledInput=0.0  OutMin=[]  OutMax=[]  OutDataType=fixdt(1, 16)  OutScaling=2^-10  DoSatur=off
  Discrete Derivative2 : simulink/Discrete/Discrete Derivative  gainval=1.0  ICPrevScaledInput=0.0  OutMin=[]  OutMax=[]  OutDataType=fixdt(1, 16)  OutScaling=2^-10  DoSatur=off
  Matrix Multiply : Product  Multiplication=Matrix(*)
  Mux : Mux  Inputs=3
  Mux1 : Mux  Inputs=2
  Mux2 : Mux  Inputs=3
  Reshape1 : Reshape  OutputDimensionality=Column vector (2-D)
  Reshape2 : Reshape  OutputDimensionality=Column vector (2-D)
  Reshape4 : Reshape  OutputDimensionality=Column vector (2-D)
  Subtract{4..8} (5 alike) : Sum  Inputs=-+
  Terminator : Terminator
  u : Outport
  wires:
  Calculate Error/1(Attitude Error) -> Mux/3
  Subtract6/1 -> Mux2/2
  Matrix Multiply/1 -> Reshape4/1
  Mux2/1 -> Reshape2/1
  Reshape4/1 -> u/1
  Mux/1 -> Reshape1/1
  Subtract5/1 -> Mux/1
  Reshape2/1 -> Mux1/2
  Mux1/1 -> Matrix Multiply/2
  Subtract7/1 -> Mux2/1
  Constant2/1 -> Matrix Multiply/1
  Subtract4/1 -> Mux/2
  Subtract8/1 -> Mux2/3
  Reshape1/1 -> Mux1/1
  Demux/2 -> Subtract4/2
  Demux/4 -> Subtract7/2
  Demux/7 -> Terminator/1
  Demux/1 -> Subtract5/2
  Data Store Read1/1 -> Demux1/1
  Discrete Derivative2/1 -> Subtract8/1
  Demux1/3 -> Calculate Error/1(Desired Attitude), Discrete Derivative2/1
  Discrete Derivative/1 -> Subtract7/1
  Demux/3 -> Calculate Error/2(Measured Attitude)
  Demux1/2 -> Discrete Derivative1/1, Subtract4/1
  Demux/6 -> Subtract8/2
  Demux/5 -> Subtract6/2
  Data Store Read2/1 -> Demux/1
  Demux1/1 -> Discrete Derivative/1, Subtract5/1
  Discrete Derivative1/1 -> Subtract6/1

== system Capstone_MPC_Final/3 - Control/Default LQR Control (RED) ==
  Action Port : ActionPort  ActionPortLabel=elseif(u1 == 2)
  Calculate Error : Subsystem
  Constant2 : Constant  Value=-K_RED
  Data Store Read1 : DataStoreRead  DataStoreName=RED_Path  IndexOptions=Index vector (dialog)  Indices=1  OutputSizes=1
  Data Store Read13 : DataStoreRead  DataStoreName=RED_Measured_States  IndexOptions=Index vector (dialog)  Indices=1  OutputSizes=1
  Demux : Demux  Outputs=[1,1,1,1,1,1,3]
  Demux1 : Demux  Outputs=3
  Discrete Derivative : simulink/Discrete/Discrete Derivative  gainval=1.0  ICPrevScaledInput=0.0  OutMin=[]  OutMax=[]  OutDataType=fixdt(1, 16)  OutScaling=2^-10  DoSatur=off
  Discrete Derivative1 : simulink/Discrete/Discrete Derivative  gainval=1.0  ICPrevScaledInput=0.0  OutMin=[]  OutMax=[]  OutDataType=fixdt(1, 16)  OutScaling=2^-10  DoSatur=off
  Discrete Derivative2 : simulink/Discrete/Discrete Derivative  gainval=1.0  ICPrevScaledInput=0.0  OutMin=[]  OutMax=[]  OutDataType=fixdt(1, 16)  OutScaling=2^-10  DoSatur=off
  Matrix Multiply : Product  Multiplication=Matrix(*)
  Mux1 : Mux  Inputs=3
  Mux2 : Mux  Inputs=2
  Mux3 : Mux  Inputs=3
  Reshape2 : Reshape  OutputDimensionality=Column vector (2-D)
  Reshape3 : Reshape  OutputDimensionality=Column vector (2-D)
  Reshape4 : Reshape  OutputDimensionality=Column vector (2-D)
  Subtract{4..8} (5 alike) : Sum  Inputs=-+
  Terminator : Terminator
  u : Outport
  wires:
  Subtract5/1 -> Mux1/1
  Mux2/1 -> Matrix Multiply/2
  Reshape3/1 -> Mux2/2
  Mux1/1 -> Reshape2/1
  Matrix Multiply/1 -> Reshape4/1
  Reshape4/1 -> u/1
  Subtract7/1 -> Mux3/1
  Reshape2/1 -> Mux2/1
  Mux3/1 -> Reshape3/1
  Constant2/1 -> Matrix Multiply/1
  Subtract4/1 -> Mux1/2
  Subtract8/1 -> Mux3/3
  Calculate Error/1(Attitude Error) -> Mux1/3
  Subtract6/1 -> Mux3/2
  Demux1/1 -> Discrete Derivative/1, Subtract5/1
  Discrete Derivative/1 -> Subtract7/1
  Demux1/3 -> Calculate Error/1(Desired Attitude), Discrete Derivative2/1
  Discrete Derivative1/1 -> Subtract6/1
  Demux/5 -> Subtract6/2
  Demux/3 -> Calculate Error/2(Measured Attitude)
  Demux/7 -> Terminator/1
  Data Store Read1/1 -> Demux1/1
  Demux/2 -> Subtract4/2
  Demux/1 -> Subtract5/2
  Demux/4 -> Subtract7/2
  Demux1/2 -> Discrete Derivative1/1, Subtract4/1
  Discrete Derivative2/1 -> Subtract8/1
  Data Store Read13/1 -> Demux/1
  Demux/6 -> Subtract8/2

== system Capstone_MPC_Final/3 - Control/Default PD (ARM) ==
  Action Port : ActionPort  ActionPortLabel=if(u1 == 1 )
  Constant7 : Constant
  Data Store Read2 : DataStoreRead  DataStoreName=ARM_Path  IndexOptions=Index vector (dialog)  Indices=1  OutputSizes=1
  Data Store Read4 : DataStoreRead  DataStoreName=isSim  IndexOptions=Index vector (dialog)  Indices=1  OutputSizes=1
  Data Store Write12 : DataStoreWrite  DataStoreName=ARM_Control_Mode  IndexOptions=Index vector (dialog)  Indices=1  OutputSizes=1
  Demux : Demux  Outputs=3
  "If 'simMode' set to '1', then this is a simulation and the dynamics will be simulated. Otherwise, this is an experiment, and the simulation will not be run." : If  IfExpression=u1 == 1
  Merge3 : Merge
  Merge4 : Merge
  Merge5 : Merge
  Mux : Mux  Inputs=3
  Passthrough for Experiment : Subsystem  TreatAsAtomicUnit=on
  Scope : Scope
  Simulated Position Controller : Subsystem  TreatAsAtomicUnit=on
  u : Outport
  wires:
  Passthrough for Experiment/3(q3_command) -> Merge5/2
  Data Store Read4/1 -> "If 'simMode' set to '1', then this is a simulation and the dynamics will be simulated. Otherwise, this is an experiment, and the simulation will not be run."/1
  Demux/3 -> Passthrough for Experiment/3(q3_desired), Simulated Position Controller/3(q3_desired)
  Simulated Position Controller/1(q1_command) -> Merge3/1
  Simulated Position Controller/3(q3_command) -> Merge5/1
  "If 'simMode' set to '1', then this is a simulation and the dynamics will be simulated. Otherwise, this is an experiment, and the simulation will not be run."/1 -> Simulated Position Controller/Action
  Demux/2 -> Passthrough for Experiment/2(q2_desired), Simulated Position Controller/2(q2_desired)
  Passthrough for Experiment/2(q2_command) -> Merge4/2
  Simulated Position Controller/2(q2_command) -> Merge4/1
  Constant7/1 -> Data Store Write12/1
  Passthrough for Experiment/1(q1_command) -> Merge3/2
  Demux/1 -> Passthrough for Experiment/1(q1_desired), Simulated Position Controller/1(q1_desired)
  "If 'simMode' set to '1', then this is a simulation and the dynamics will be simulated. Otherwise, this is an experiment, and the simulation will not be run."/2 -> Passthrough for Experiment/Action
  Merge3/1 -> Mux/1
  Merge4/1 -> Mux/2
  Merge5/1 -> Mux/3
  Mux/1 -> Scope/1, u/1
  Data Store Read2/1 -> Demux/1

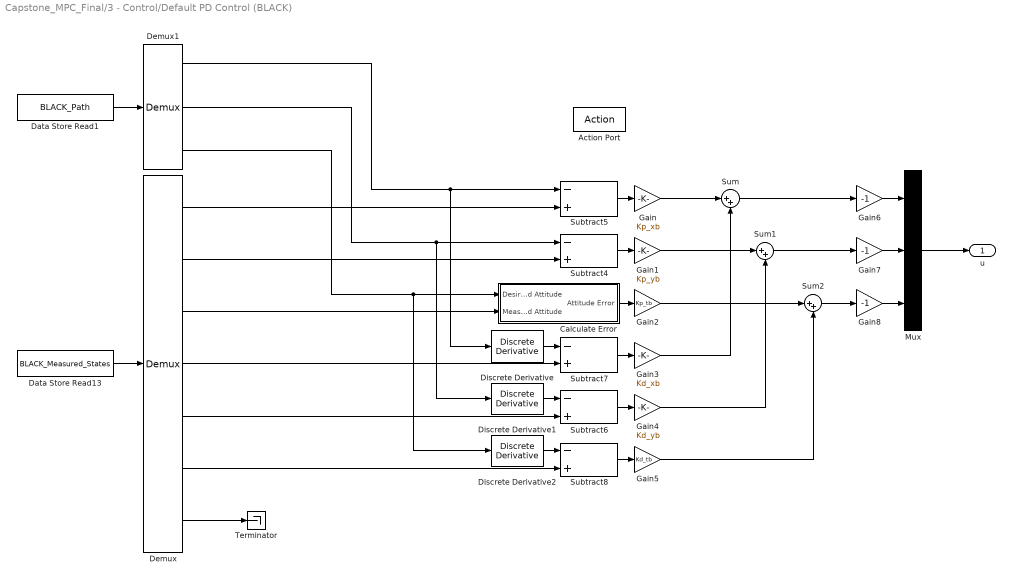
== system Capstone_MPC_Final/3 - Control/Default PD Control (BLACK) ==
  Action Port : ActionPort  ActionPortLabel=if(u1 == 1 )
  Calculate Error : Subsystem
  Data Store Read1 : DataStoreRead  DataStoreName=BLACK_Path  IndexOptions=Index vector (dialog)  Indices=1  OutputSizes=1
  Data Store Read13 : DataStoreRead  DataStoreName=BLACK_Measured_States  IndexOptions=Index vector (dialog)  Indices=1  OutputSizes=1
  Demux : Demux  Outputs=[1,1,1,1,1,1,3]
  Demux1 : Demux  Outputs=3
  Discrete Derivative : simulink/Discrete/Discrete Derivative  gainval=1.0  ICPrevScaledInput=0.0  OutMin=[]  OutMax=[]  OutDataType=fixdt(1, 16)  OutScaling=2^-10  DoSatur=off
  Discrete Derivative1 : simulink/Discrete/Discrete Derivative  gainval=1.0  ICPrevScaledInput=0.0  OutMin=[]  OutMax=[]  OutDataType=fixdt(1, 16)  OutScaling=2^-10  DoSatur=off
  Discrete Derivative2 : simulink/Discrete/Discrete Derivative  gainval=1.0  ICPrevScaledInput=0.0  OutMin=[]  OutMax=[]  OutDataType=fixdt(1, 16)  OutScaling=2^-10  DoSatur=off
  Gain : Gain  Gain=Kp_xb
  Gain1 : Gain  Gain=Kp_yb
  Gain2 : Gain  Gain=Kp_tb
  Gain3 : Gain  Gain=Kd_xb
  Gain4 : Gain  Gain=Kd_yb
  Gain5 : Gain  Gain=Kd_tb
  Gain6 : Gain  Gain=-1
  Gain7 : Gain  Gain=-1
  Gain8 : Gain  Gain=-1
  Mux : Mux  Inputs=3
  Subtract{4..8} (5 alike) : Sum  Inputs=-+
  Sum : Sum  Inputs=|++
  Sum1 : Sum  Inputs=|++
  Sum2 : Sum  Inputs=|++
  Terminator : Terminator
  u : Outport
  wires:
  Demux/6 -> Subtract8/2
  Subtract8/1 -> Gain5/1
  Gain8/1 -> Mux/3
  Discrete Derivative2/1 -> Subtract8/1
  Gain1/1 -> Sum1/1
  Subtract5/1 -> Gain/1
  Discrete Derivative1/1 -> Subtract6/1
  Subtract6/1 -> Gain4/1
  Demux/2 -> Subtract4/2
  Demux/1 -> Subtract5/2
  Sum1/1 -> Gain7/1
  Demux/4 -> Subtract7/2
  Demux1/3 -> Calculate Error/1(Desired Attitude), Discrete Derivative2/1
  Sum/1 -> Gain6/1
  Subtract4/1 -> Gain1/1
  Demux/3 -> Calculate Error/2(Measured Attitude)
  Subtract7/1 -> Gain3/1
  Gain3/1 -> Sum/2
  Mux/1 -> u/1
  Gain4/1 -> Sum1/2
  Demux1/2 -> Discrete Derivative1/1, Subtract4/1
  Gain/1 -> Sum/1
  Demux/5 -> Subtract6/2
  Gain5/1 -> Sum2/2
  Discrete Derivative/1 -> Subtract7/1
  Demux1/1 -> Discrete Derivative/1, Subtract5/1
  Sum2/1 -> Gain8/1
  Calculate Error/1(Attitude Error) -> Gain2/1
  Gain7/1 -> Mux/2
  Gain6/1 -> Mux/1
  Gain2/1 -> Sum2/1
  Data Store Read13/1 -> Demux/1
  Demux/7 -> Terminator/1
  Data Store Read1/1 -> Demux1/1
